simulink model "mpc_func"  (R2021a)
settings: Solver=VariableStepAuto  StartTime=0.0  StopTime=0.01  RelTol=1e-1
settings Model: Creator=davidrico  LastModifiedBy=davidrico

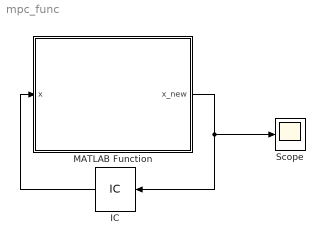
== system mpc_func ==
  IC : InitialCondition  Value=[10; 0]
  MATLAB Function : MATLAB Function  TreatAsAtomicUnit=on
  Scope : Scope
  wires:
  MATLAB Function/1(x_new) -> IC/1, Scope/1
  IC/1 -> MATLAB Function/1(x)

== matlab function mpc_func/MATLAB Function ==
  data: x input; x_new output
function x_new = fcn(x)
x_new = zeros(2, 1);
A = [1 1; 0 1];
B = [0; 1];

Q = [1 0; 0 0];
Q_spec = blkdiag(Q, Q, Q);
B_spec = [0 0 0; 0 0 0; 0 0 0; 1 0 0; 1 0 0; 1 1 0];
R = 1/10;
R_spec = blkdiag(R, R, R);
A_spec = [eye(2); A; A^2];

H = 2*(B_spec'*Q_spec*B_spec + R_spec);
A_constraints = [1 0 0; -1 0 0; 0 1 0; 0 -1 0; 0 0 1; 0 0 -1];
b_constraints = ones(6, 1);

f = 2*x'*A_spec'*Q_spec*B_spec;
coder.extrinsic('quadprog');
min_of_J = quadprog(H,f,A_constraints,b_constraints);
u = 0;
u = min_of_J(1,1);
x_new = A*x + B*u;
